simulink model "Proj4_sim"  (R2024b)
settings: Solver=VariableStepAuto  StartTime=0.0  StopTime=6000  RelTol=1e-3
values from neighbouring files (symbols this model uses):
  track_elevation_s = s_vals    [Proj4_track.m]
  track_elevation_z = elevation_profile    [Proj4_track.m]
undefined symbols (not defined in the file or in its folder): carData, datBat, datCar, datMotor, K_d, K_i, K_p
libraries: slpidlib x1, simulink x1
settings Model: NumberOfSteps=50  Creator=dxego  LastModifiedBy=jacobcody
settings RTWCC: GPUComputeCapability=3.5

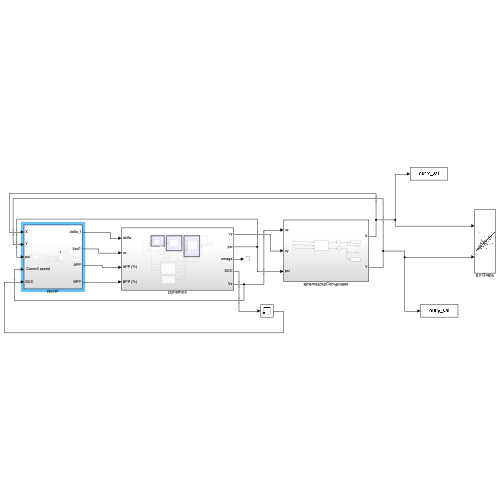
[thumbnail: Simulink's stored preview of the top-level diagram]
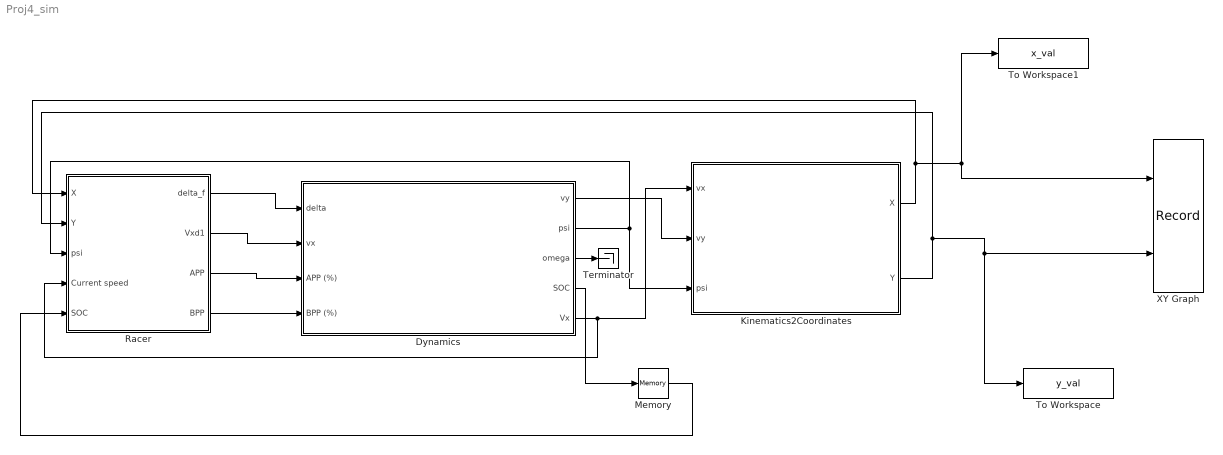
== system Proj4_sim ==
  Dynamics : Subsystem
  Kinematics2Coordinates : Subsystem
  Memory : Memory
  Racer : Subsystem
  Terminator : Terminator
  To Workspace : ToWorkspace  VariableName=y_val  SaveFormat=Timeseries  SampleTime=-1
  To Workspace1 : ToWorkspace  VariableName=x_val  SaveFormat=Timeseries  SampleTime=-1
  XY Graph : Record  FileSettingsInternal="{\"entries\":[{\"content\":{\"excelSettings\":{\"content\":{},\"type\":\"Streamout.ExcelSettings\"}},\"type\":\"Streamout.FileSettingStorage\",\"uuid\":\"\"}],\"packageUris\":[\"http:\\/\\/schema.mathworks.com\\/mf0\\/streamout_blocks\\/R2020a\"],\"version\":\"1.0\"}"  Layout=[1 1]  SignalsInternal="{\"entries\":[{\"content\":{\"signals\":[{\"content\":{\"blockPath\":[],\"dimensions\":[1],\"domain\":\"\",\"lineColor\":\"#ff13a6\",\"lineWidth\":2,\"port\":1,\"sid\":[\"\"],\"signalID\":1,\"signalName\":\"Kinematics2Coordinates:1\"},\"type\":\"RecordBlkView.Signal\",\"uuid\":\"\"},{\"content\":{\"blockPath\":[],\"dimensions\":[1],\"domain\":\"\",\"lineColor\":\"#139fff\",\"plots\":[ 1 ],\"port\":2,\"sid\":[\"\"],\"signalID\":2,\"signalName\":\"Kinematics2Coordinates:2\"},\"type\":\"RecordBlkView.Signal\",\"uuid\":\"\"}]},\"type\":\"RecordBlkView.InputSignals\",\"uuid\":\"\"}],\"packageUris\":[\"http:\\/\\/schema.mathworks.com\\/mf0\\/streamout_blocks\\/R2020a\"],\"version\":\"1.0\"}"  VisualizationBindings="{\"xyplotplugin\":{\"info\":[{\"series\":[{\"bindingParametersList\":[{\"parameter\":\"Y-Axis\",\"signalID\":2,\"signalName\":\"Kinematics2Coordinates:2\"}],\"seriesID\":0}],\"subplotID\":1}]}}"  CompatibilityTag=XY
  wires:
  Dynamics/1(vy) -> Kinematics2Coordinates/2(vy)
  Kinematics2Coordinates/1(X) -> Racer/1(X), To Workspace1/1, XY Graph/1
  Kinematics2Coordinates/2(Y) -> Racer/2(Y), To Workspace/1, XY Graph/2
  Racer/2(Vxd1) -> Dynamics/2(vx)
  Racer/1(delta_f) -> Dynamics/1(delta)
  Dynamics/2(psi) -> Kinematics2Coordinates/3(psi), Racer/3(psi)
  Dynamics/3(omega) -> Terminator/1
  Racer/3(APP) -> Dynamics/3(APP (%))
  Racer/4(BPP) -> Dynamics/4(BPP (%))
  Dynamics/5(Vx) -> Kinematics2Coordinates/1(vx), Racer/4(" Current speed")
  Memory/1 -> Racer/5("SOC ")
  Dynamics/4(SOC) -> Memory/1

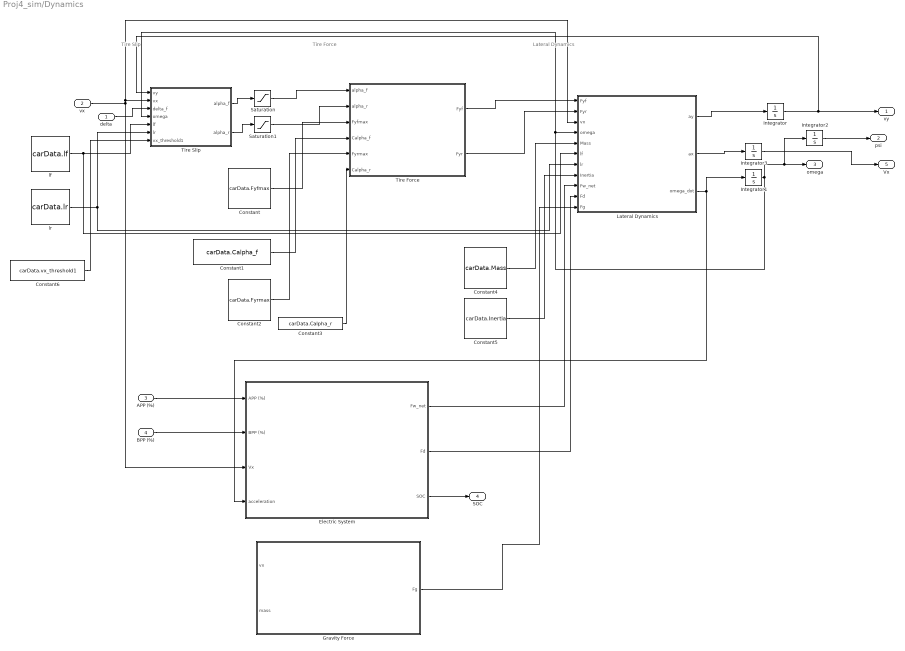
== system Proj4_sim/Dynamics ==
  note: Tire Slip
  note: Tire Force
  note: Lateral Dynamics
  delta : Inport
  vx : Inport  Port=2
  APP (%) : Inport  Port=3
  BPP (%) : Inport  Port=4
  Constant : Constant  Value=carData.Fyfmax
  Constant1 : Constant  Value=carData.Calpha_f
  Constant2 : Constant  Value=carData.Fyrmax
  Constant3 : Constant  Value=carData.Calpha_r
  Constant4 : Constant  Value=carData.Mass
  Constant5 : Constant  Value=carData.Inertia
  Constant6 : Constant  Value=carData.vx_threshold1
  Electric System : Subsystem
  Gravity Force : Subsystem
  Integrator : Integrator  InitialCondition=carData.init.vy0
  Integrator1 : Integrator  InitialCondition=carData.init.omega0
  Integrator2 : Integrator  InitialCondition=carData.init.psi0  WrappedStateUpperValue=2*pi  WrappedStateLowerValue=0
  Integrator3 : Integrator  InitialCondition=.01  IgnoreLimit=on
  Lateral Dynamics : MATLAB Function  TreatAsAtomicUnit=on
  Saturation : Saturate  UpperLimit=carData.maxAlpha  LowerLimit=-carData.maxAlpha
  Saturation1 : Saturate  UpperLimit=carData.maxAlpha  LowerLimit=-carData.maxAlpha
  Tire Force : MATLAB Function  TreatAsAtomicUnit=on
  "Tire Slip " : MATLAB Function  TreatAsAtomicUnit=on
  lf : Constant  Value=carData.lf
  lr : Constant  Value=carData.lr
  vy : Outport
  psi : Outport  Port=2
  omega : Outport  Port=3
  SOC : Outport  Port=4
  Vx : Outport  Port=5
  wires:
  Lateral Dynamics/1(ay) -> Integrator/1
  Integrator/1 -> "Tire Slip "/1(vy), vy/1
  Lateral Dynamics/3(omega_dot) -> Integrator1/1, Electric System/4(acceleration)
  Integrator1/1 -> Integrator2/1, omega/1, "Tire Slip "/4(omega), Lateral Dynamics/4(omega)
  "Tire Slip "/1(alpha_f) -> Saturation/1
  Saturation/1 -> Tire Force/1(alpha_f)
  Saturation1/1 -> Tire Force/2(alpha_r)
  vx/1 -> Lateral Dynamics/3(vx), "Tire Slip "/2(vx), Electric System/3(Vx)
  delta/1 -> "Tire Slip "/3(delta_f)
  Integrator2/1 -> psi/1
  "Tire Slip "/2(alpha_r) -> Saturation1/1
  Tire Force/1(Fyf) -> Lateral Dynamics/1(Fyf)
  Tire Force/2(Fyr) -> Lateral Dynamics/2(Fyr)
  lf/1 -> Lateral Dynamics/6(lf), "Tire Slip "/5(lf)
  lr/1 -> Lateral Dynamics/7(lr), "Tire Slip "/6(lr)
  Constant/1 -> Tire Force/3(Fyfmax)
  Constant1/1 -> Tire Force/4(Calpha_f)
  Constant2/1 -> Tire Force/5(Fyrmax)
  Constant3/1 -> Tire Force/6(Calpha_r)
  Constant4/1 -> Lateral Dynamics/5(Mass)
  Constant5/1 -> Lateral Dynamics/8(Inertia)
  Constant6/1 -> "Tire Slip "/7(vx_threshold1)
  APP (%)/1 -> Electric System/1(APP (%))
  BPP (%)/1 -> Electric System/2(BPP (%))
  Electric System/3(SOC) -> SOC/1
  Lateral Dynamics/2(ax) -> Integrator3/1
  Integrator3/1 -> Vx/1
  Electric System/2(Fd) -> Lateral Dynamics/10(Fd)
  Gravity Force/1(Fg) -> Lateral Dynamics/11(Fg)
  Electric System/1(Fw_net) -> Lateral Dynamics/9(Fw_net)

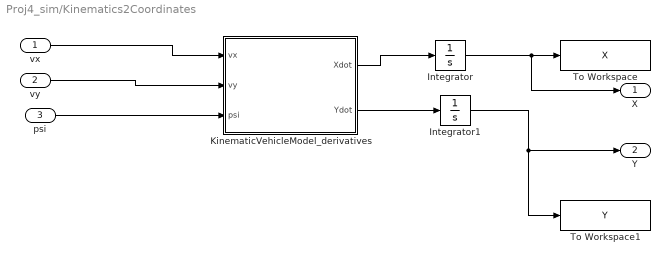
== system Proj4_sim/Kinematics2Coordinates ==
  vx : Inport
  vy : Inport  Port=2
  psi : Inport  Port=3
  Integrator : Integrator  InitialCondition=carData.init.X0
  Integrator1 : Integrator  InitialCondition=carData.init.Y0
  KinematicVehicleModel_derivatives : MATLAB Function  TreatAsAtomicUnit=on
  To Workspace : ToWorkspace  VariableName=X  SaveFormat=Timeseries  SampleTime=-1
  To Workspace1 : ToWorkspace  VariableName=Y  SaveFormat=Timeseries  SampleTime=-1
  X : Outport
  Y : Outport  Port=2
  wires:
  Integrator/1 -> X/1, To Workspace/1
  Integrator1/1 -> To Workspace1/1, Y/1
  vx/1 -> KinematicVehicleModel_derivatives/1(vx)
  vy/1 -> KinematicVehicleModel_derivatives/2(vy)
  psi/1 -> KinematicVehicleModel_derivatives/3(psi)
  KinematicVehicleModel_derivatives/1(Xdot) -> Integrator/1
  KinematicVehicleModel_derivatives/2(Ydot) -> Integrator1/1

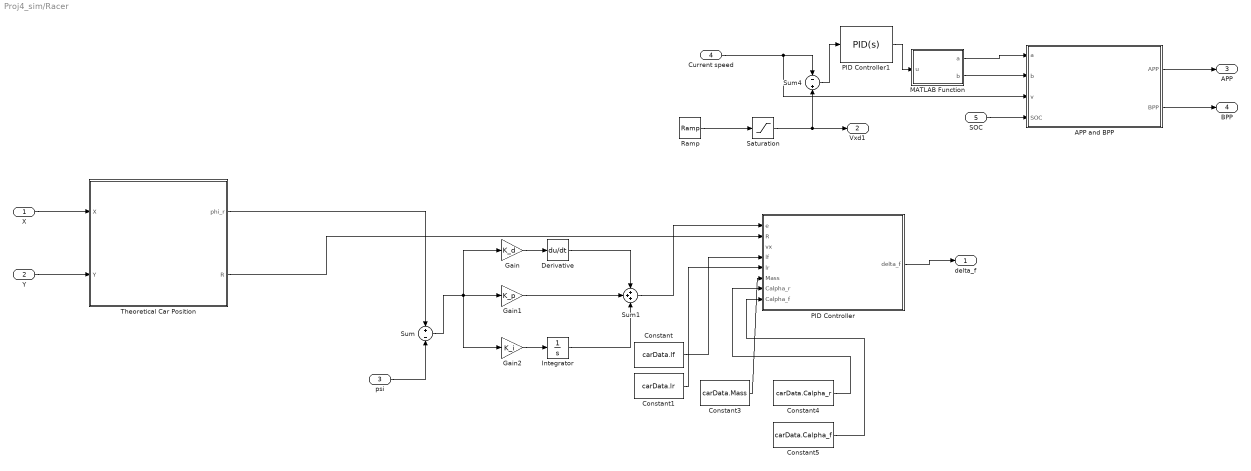
== system Proj4_sim/Racer ==
  X : Inport
  Y : Inport  Port=2
  psi : Inport  Port=3
  " Current speed" : Inport  Port=4
  "SOC " : Inport  Port=5
  "APP and BPP " : MATLAB Function  TreatAsAtomicUnit=on
  Constant : Constant  Value=carData.lf
  Constant1 : Constant  Value=carData.lr
  Constant3 : Constant  Value=carData.Mass
  Constant4 : Constant  Value=carData.Calpha_r
  Constant5 : Constant  Value=carData.Calpha_f
  Derivative : Derivative
  Gain : Gain  Gain=K_d
  Gain1 : Gain  Gain=K_p
  Gain2 : Gain  Gain=K_i
  Integrator : Integrator
  MATLAB Function : MATLAB Function  TreatAsAtomicUnit=on
  PID Controller : MATLAB Function  TreatAsAtomicUnit=on
  PID Controller1 : slpidlib/PID Controller  Controller=PID  Form=Parallel  TimeDomain=Continuous-time  UseExternalTs=off  SampleTime=-1  IntegratorMethod=Forward Euler  FilterMethod=Forward Euler  ControllerParametersSource=internal  P=2  I=0.8  UseKiTs=off  D=0  UseExternalDerivativeSource=off  N=100  UseFilter=on  TunerSelectOption=Transfer Function Based (PID Tuner App)  InitialConditionSource=internal  InitialConditionForIntegrator=0  InitialConditionForFilter=0  DifferentiatorICPrevScaledInput=0  ExternalReset=none  TrackingMode=off  Kt=1  LimitOutput=off  SatLimitsSource=internal  UpperSaturationLimit=inf  LowerSaturationLimit=-inf  LinearizeAsGain=on  AntiWindupMode=none  Kb=1  LimitIntegrator=off  UpperIntegratorSaturationLimit=inf  LowerIntegratorSaturationLimit=-inf  POutMin=[]  POutMax=[]  IOutMin=[]  IOutMax=[]  DOutMin=[]  DOutMax=[]  NOutMin=[]  NOutMax=[]  SumOutMin=[]  SumOutMax=[]  SaturationOutMin=[]  SaturationOutMax=[]  PParamMin=[]  PParamMax=[]  IParamMin=[]  IParamMax=[]  DParamMin=[]  DParamMax=[]  NParamMin=[]  NParamMax=[]  KbParamMin=[]  KbParamMax=[]  KtParamMin=[]  KtParamMax=[]  KbOutMin=[]  KbOutMax=[]  KtOutMin=[]  KtOutMax=[]  IntegratorOutMin=[]  IntegratorOutMax=[]  FilterOutMin=[]  FilterOutMax=[]  SumI1OutMin=[]  SumI1OutMax=[]  SumI2OutMin=[]  SumI2OutMax=[]  SumI3OutMin=[]  SumI3OutMax=[]  SumI4OutMin=[]  SumI4OutMax=[]  SumDOutMin=[]  SumDOutMax=[]  DifferentiatorOutMin=[]  DifferentiatorOutMax=[]  FilterDiffOutCoefMin=[]  FilterDiffOutCoefMax=[]  ReciprocalOutMin=[]  ReciprocalOutMax=[]  SumDenOutMin=[]  SumDenOutMax=[]  SumNumOutMin=[]  SumNumOutMax=[]  DivideOutMin=[]  DivideOutMax=[]  UdiffTsProdOutMin=[]  UdiffTsProdOutMax=[]  NTsProdOutMin=[]  NTsProdOutMax=[]  UintegralTsProdOutMin=[]  UintegralTsProdOutMax=[]  UngainTsProdOutMin=[]  UngainTsProdOutMax=[]  ClampingZeroOutDataTypeStr=Inherit: Inherit via back propagation  ClampingZeroOutMin=[]  ClampingZeroOutMax=[]  FilterDenConstantOutDataTypeStr=Inherit: Inherit via back propagation  FilterDenConstantOutMin=[]  FilterDenConstantOutMax=[]  PCopyOutDataTypeStr=Inherit: Inherit via back propagation  PCopyOutMin=[]  PCopyOutMax=[]  NCopyOutDataTypeStr=Inherit: Inherit via back propagation  NCopyOutMin=[]  NCopyOutMax=[]  IntegratorContinuousStateAttributes=''  IntegratorStateMustResolveToSignalObject=off  IntegratorRTWStateStorageClass=Auto  FilterContinuousStateAttributes=''  FilterStateMustResolveToSignalObject=off  FilterRTWStateStorageClass=Auto  ParallelPVariant=InternalParameters  IdealPVariant=Disabled  IVariant=InternalParameters  DVariant=InternalParameters  IntegratorVariant=Continuous  SatVariant=Disabled  AWVariant=Passthrough  PCopyVariant=Disabled  TRVariant=Disabled  FdbkBlocksVariant=Forward  IdealPFdbkVariant=Disabled  SatFdbkVariant=Disabled  DerivativeFilterVariant=ContFilter  NVariant=InternalParameters  NCopyVariant=Disabled  FilterICVariant=InternalICsFilter  IntegratorICVariant=InternalICs  ExternalResetVariant=Disabled  TRSumVariant=Passthrough  SumFdbkVariant=Disabled  SumVariant=Sum_PID  TsampFilterVariant=InternalTs  TsampNgainVariant=Passthrough  TsampIntegralVariant=Disabled_SignalSpec  ExternalSaturationOutDataTypeStr=Inherit: Same as second input  DerivativeSourceVariant=ErrorSignal  PreIntVariant=InternalPreInt
  Ramp : simulink/Sources/Ramp  slope=2.5  start=0  InitialOutput=0
  Saturation : Saturate  UpperLimit=10  LowerLimit=0
  Sum : Sum  Inputs=+-
  Sum1 : Sum  Inputs=+++
  Sum4 : Sum  Inputs=-+
  Theoretical Car Position : MATLAB Function  TreatAsAtomicUnit=on
  delta_f : Outport
  Vxd1 : Outport  Port=2
  APP : Outport  Port=3
  BPP : Outport  Port=4
  wires:
  Y/1 -> Theoretical Car Position/2(Y)
  psi/1 -> Sum/2
  Gain/1 -> Derivative/1
  Gain2/1 -> Integrator/1
  Sum/1 -> Gain2/1, Gain/1, Gain1/1
  Derivative/1 -> Sum1/1
  Gain1/1 -> Sum1/2
  Integrator/1 -> Sum1/3
  Sum1/1 -> PID Controller/1(e)
  X/1 -> Theoretical Car Position/1(X)
  Constant/1 -> PID Controller/4(lf)
  Constant1/1 -> PID Controller/5(lr)
  Constant3/1 -> PID Controller/6(Mass)
  Constant4/1 -> PID Controller/7(Calpha_r)
  Constant5/1 -> PID Controller/8(Calpha_f)
  Theoretical Car Position/1(phi_r) -> Sum/1
  Theoretical Car Position/2(R) -> PID Controller/2(R)
  PID Controller/1(delta_f) -> delta_f/1
  Ramp/1 -> Saturation/1
  "APP and BPP "/1(APP) -> APP/1
  "APP and BPP "/2(BPP) -> BPP/1
  "SOC "/1 -> "APP and BPP "/4(SOC)
  " Current speed"/1 -> "APP and BPP "/3(v), Sum4/1
  Saturation/1 -> Vxd1/1, Sum4/2
  Sum4/1 -> PID Controller1/1
  PID Controller1/1 -> MATLAB Function/1(u)
  MATLAB Function/1(a) -> "APP and BPP "/1(a)
  MATLAB Function/2(b) -> "APP and BPP "/2(b)

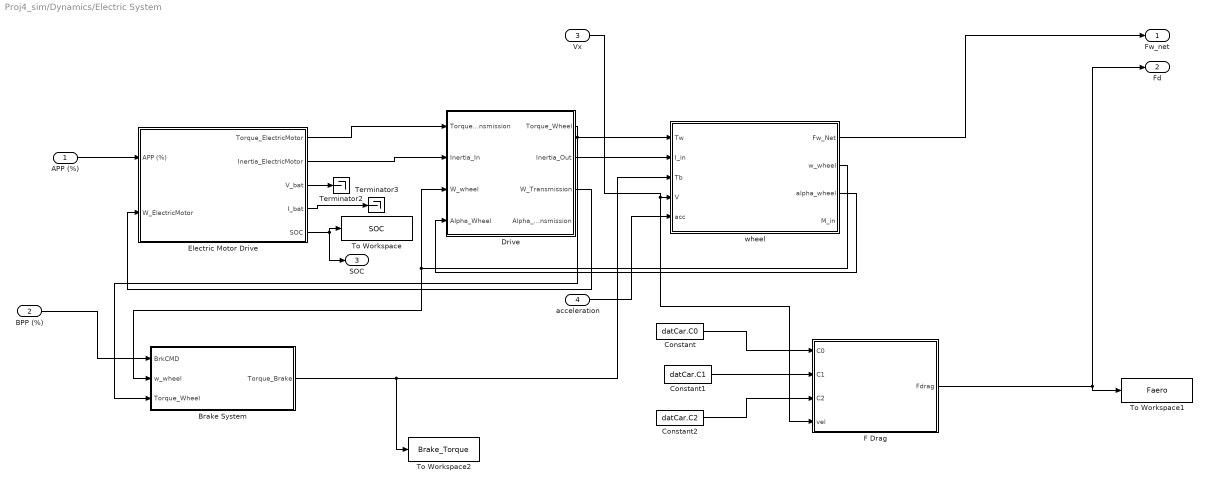
== system Proj4_sim/Dynamics/Electric System ==
  APP (%) : Inport
  BPP (%) : Inport  Port=2
  Vx : Inport  Port=3
  acceleration : Inport  Port=4
  "Brake System " : Subsystem
  Constant : Constant  Value=datCar.C0
  Constant1 : Constant  Value=datCar.C1
  Constant2 : Constant  Value=datCar.C2
  Drive : Subsystem
  Electric Motor Drive : Subsystem
  F Drag : MATLAB Function  TreatAsAtomicUnit=on
  Terminator2 : Terminator
  Terminator3 : Terminator
  To Workspace : ToWorkspace  VariableName=SOC  SaveFormat=Timeseries  SampleTime=-1
  To Workspace1 : ToWorkspace  VariableName=Faero  SaveFormat=Timeseries  SampleTime=-1
  To Workspace2 : ToWorkspace  VariableName=Brake_Torque  SaveFormat=Timeseries  SampleTime=-1
  "wheel " : Subsystem
  Fw_net : Outport
  Fd : Outport  Port=2
  SOC : Outport  Port=3
  wires:
  Drive/2(Inertia_Out) -> "wheel "/2(I_in)
  Vx/1 -> F Drag/4(vel), "wheel "/4(V)
  Drive/1(Torque_Wheel) -> "Brake System "/3(Torque_Wheel), "wheel "/1(Tw)
  APP (%)/1 -> Electric Motor Drive/1(APP (%))
  Electric Motor Drive/1(Torque_ElectricMotor) -> Drive/1(Torque_Transmission)
  Electric Motor Drive/2(Inertia_ElectricMotor) -> Drive/2(Inertia_In)
  Electric Motor Drive/3(V_bat) -> Terminator2/1
  Electric Motor Drive/4(I_bat) -> Terminator3/1
  Electric Motor Drive/5(SOC) -> To Workspace/1, SOC/1
  acceleration/1 -> "wheel "/5(acc)
  "wheel "/1(Fw_Net) -> Fw_net/1
  F Drag/1(Fdrag) -> To Workspace1/1, Fd/1
  BPP (%)/1 -> "Brake System "/1("BrkCMD ")
  "wheel "/3(alpha_wheel) -> Drive/4(Alpha_Wheel)
  "wheel "/2(w_wheel) -> Drive/3(W_wheel), "Brake System "/2("w_wheel ")
  Constant/1 -> F Drag/1(C0)
  Constant1/1 -> F Drag/2(C1)
  Constant2/1 -> F Drag/3(C2)
  "Brake System "/1("Torque_Brake ") -> To Workspace2/1, "wheel "/3(Tb)
  Drive/3(W_Transmission) -> Electric Motor Drive/2(W_ElectricMotor)

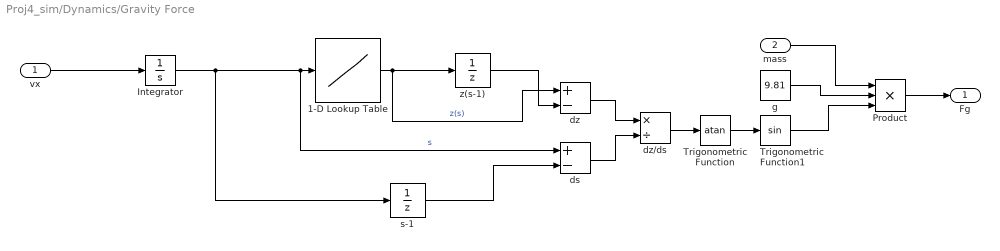
== system Proj4_sim/Dynamics/Gravity Force ==
  vx : Inport
  mass : Inport  Port=2
  1-D Lookup Table : Lookup_n-D  NumberOfTableDimensions=1  BreakpointsForDimension1=track_elevation_s  Table=track_elevation_z  InternalRulePriority=Speed  RndMeth=Simplest
  Integrator : Integrator
  Product : Product  Inputs=3
  Trigonometric Function : Trigonometry  Operator=atan
  Trigonometric Function1 : Trigonometry
  ds : Sum  Inputs=+-
  dz : Sum  Inputs=+-
  dz/ds : Product  Inputs=*/
  g : Constant  Value=9.81
  s-1 : UnitDelay  SampleTime=-1  HasFrameUpgradeWarning=on
  z(s-1) : UnitDelay  SampleTime=-1  HasFrameUpgradeWarning=on
  Fg : Outport
  wires:
  vx/1 -> Integrator/1
  Integrator/1 -> s-1/1, ds/1, 1-D Lookup Table/1  "s"
  1-D Lookup Table/1 -> z(s-1)/1, dz/1  "z(s)"
  z(s-1)/1 -> dz/2
  dz/1 -> dz/ds/1
  ds/1 -> dz/ds/2
  dz/ds/1 -> Trigonometric Function/1
  Trigonometric Function/1 -> Trigonometric Function1/1
  mass/1 -> Product/1
  g/1 -> Product/2
  Trigonometric Function1/1 -> Product/3
  Product/1 -> Fg/1
  s-1/1 -> ds/2

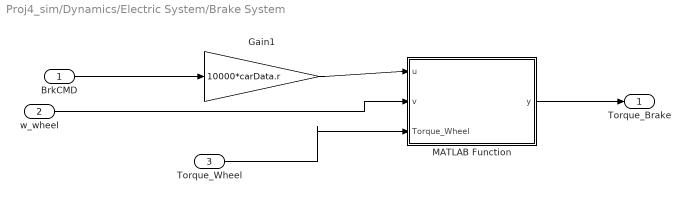
== system Proj4_sim/Dynamics/Electric System/Brake System  ==
  "BrkCMD " : Inport
  "w_wheel " : Inport  Port=2
  Torque_Wheel : Inport  Port=3
  Gain1 : Gain  Gain=10000*carData.r
  MATLAB Function : MATLAB Function  TreatAsAtomicUnit=on
  "Torque_Brake " : Outport  VectorParamsAs1DForOutWhenUnconnected=off
  wires:
  "BrkCMD "/1 -> Gain1/1
  Gain1/1 -> MATLAB Function/1(u)
  "w_wheel "/1 -> MATLAB Function/2(v)
  MATLAB Function/1(y) -> "Torque_Brake "/1
  Torque_Wheel/1 -> MATLAB Function/3(Torque_Wheel)

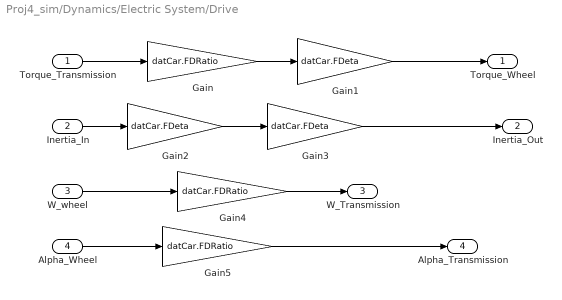
== system Proj4_sim/Dynamics/Electric System/Drive ==
  Torque_Transmission : Inport
  Inertia_In : Inport  Port=2
  W_wheel : Inport  Port=3
  Alpha_Wheel : Inport  Port=4
  Gain : Gain  Gain=datCar.FDRatio
  Gain1 : Gain  Gain=datCar.FDeta
  Gain2 : Gain  Gain=datCar.FDeta
  Gain3 : Gain  Gain=datCar.FDeta
  Gain4 : Gain  Gain=datCar.FDRatio
  Gain5 : Gain  Gain=datCar.FDRatio
  Torque_Wheel : Outport
  Inertia_Out : Outport  Port=2
  W_Transmission : Outport  Port=3
  Alpha_Transmission : Outport  Port=4
  wires:
  Torque_Transmission/1 -> Gain/1
  Gain/1 -> Gain1/1
  Gain1/1 -> Torque_Wheel/1
  Inertia_In/1 -> Gain2/1
  Gain2/1 -> Gain3/1
  Gain3/1 -> Inertia_Out/1
  W_wheel/1 -> Gain4/1
  Gain4/1 -> W_Transmission/1
  Alpha_Wheel/1 -> Gain5/1
  Gain5/1 -> Alpha_Transmission/1

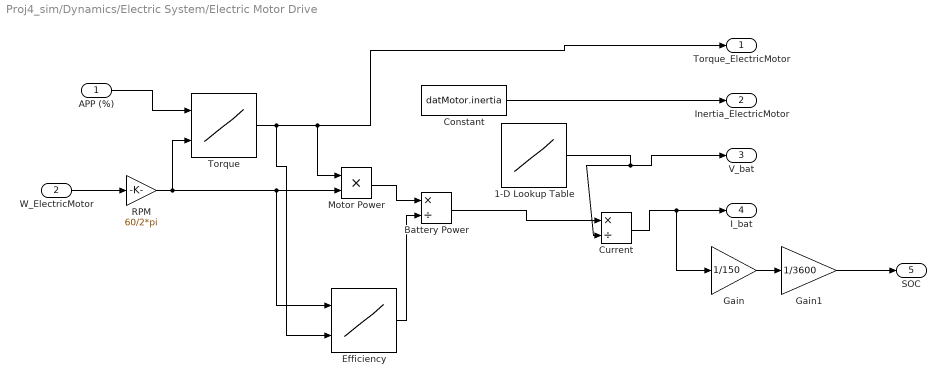
== system Proj4_sim/Dynamics/Electric System/Electric Motor Drive ==
  APP (%) : Inport
  W_ElectricMotor : Inport  Port=2
  1-D Lookup Table : Lookup_n-D  NumberOfTableDimensions=1  BreakpointsForDimension1=datBat.SOC  Table=datBat.OCV * datBat.numSeries  InternalRulePriority=Speed  RndMeth=Simplest
  Battery Power : Product  Inputs=*/
  Constant : Constant  Value=datMotor.inertia
  Current : Product  Inputs=*/
  Efficiency : Lookup_n-D  BreakpointsForDimension1=datMotor.eta_torque  BreakpointsForDimension2=datMotor.eta_speed  Table=datMotor.eta_val  InternalRulePriority=Speed  RndMeth=Simplest
      settings: InputPortMap=u0,u1
  Gain : Gain  Gain=1/150
  Gain1 : Gain  Gain=1/3600
  Motor Power : Product
  RPM : Gain  Gain=60/2*pi
  Torque : Lookup_n-D  BreakpointsForDimension1=[0,25,50,75,100]  BreakpointsForDimension2=datMotor.rpm  Table=datMotor.maxtorque  InternalRulePriority=Speed  RndMeth=Simplest
      settings: InputPortMap=u0,u1
  Torque_ElectricMotor : Outport
  Inertia_ElectricMotor : Outport  Port=2
  V_bat : Outport  Port=3
  I_bat : Outport  Port=4
  SOC : Outport  Port=5
  wires:
  Battery Power/1 -> Current/1
  1-D Lookup Table/1 -> Current/2, V_bat/1
  W_ElectricMotor/1 -> RPM/1
  APP (%)/1 -> Torque/1
  Constant/1 -> Inertia_ElectricMotor/1
  Torque/1 -> Efficiency/2, Torque_ElectricMotor/1, Motor Power/1
  Motor Power/1 -> Battery Power/1
  Efficiency/1 -> Battery Power/2
  RPM/1 -> Efficiency/1, Motor Power/2, Torque/2
  Current/1 -> Gain/1, I_bat/1
  Gain/1 -> Gain1/1
  Gain1/1 -> SOC/1

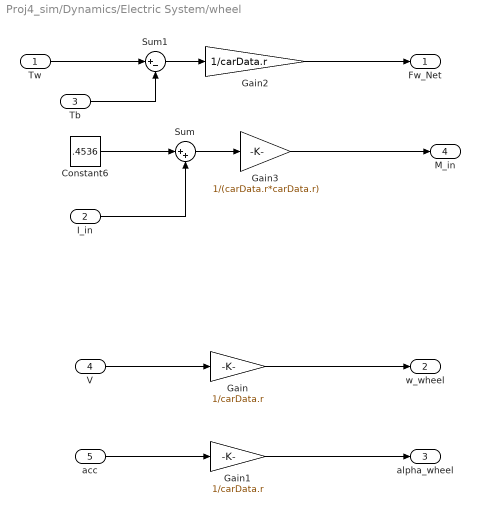
== system Proj4_sim/Dynamics/Electric System/wheel  ==
  Tw : Inport
  I_in : Inport  Port=2
  Tb : Inport  Port=3
  V : Inport  Port=4
  acc : Inport  Port=5
  Constant6 : Constant  Value=.4536
  Gain : Gain  Gain=1/carData.r
  Gain1 : Gain  Gain=1/carData.r
  Gain2 : Gain  Gain=1/carData.r
  Gain3 : Gain  Gain=1/(carData.r*carData.r)
  Sum : Sum  Inputs=|++
  Sum1 : Sum  Inputs=|+-
  Fw_Net : Outport
  w_wheel : Outport  Port=2
  alpha_wheel : Outport  Port=3
  M_in : Outport  Port=4
  wires:
  Gain/1 -> w_wheel/1
  V/1 -> Gain/1
  acc/1 -> Gain1/1
  Gain1/1 -> alpha_wheel/1
  Gain2/1 -> Fw_Net/1
  Constant6/1 -> Sum/1
  I_in/1 -> Sum/2
  Sum/1 -> Gain3/1
  Gain3/1 -> M_in/1
  Tw/1 -> Sum1/1
  Tb/1 -> Sum1/2
  Sum1/1 -> Gain2/1

== matlab function Proj4_sim/Racer/PID Controller ==
  data: e input; delta_f output; R input; vx input; lf input; lr input; Mass input; Calpha_r input; Calpha_f input
function delta_f = fcn(e, R, vx, lf, lr, Mass, Calpha_r, Calpha_f)
L = lr + lf;
if R ~= 0
    delta_f = e + (L/R)+((Mass/(L*R))*((lr/Calpha_r)-(lf/Calpha_f))*(vx^2));
else
    delta_f = e;

end

== matlab function Proj4_sim/Racer/APP and BPP  ==
  data: a input; b input; APP output; BPP output; v input; SOC input
function [APP, BPP] = fcn(a, b, v, SOC)

mph2mps = 1600/3600; % mph to m/s conversion
V_low = 5 * mph2mps;   
V_high = 25 * mph2mps; 

%Initialize
APP = 0;
BPP = 0;

if b > 0 %If braking is requested
    if v <= V_low
        FrictionPercent = 1; %100% friction
    elseif v < V_high
        FrictionPercent = 1 - 0.95 * (v - V_low) / (V_high - V_low);
    else
        FrictionPercent = 0.05; %5% friction
    end

    RegenPercent = 1 - FrictionPercent;

    if SOC <= 0.1
        RegenPercent = 0;
        FrictionPercent = 1;
    end
    APP = a + b * RegenPercent; %Add regen to throttle
    BPP = b * FrictionPercent;  %Only friction goes to brake pedal

else
    %No braking, normal acceleration
    APP = a;
    BPP = 0;
end

end

== matlab function Proj4_sim/Racer/MATLAB Function ==
  data: u input; a output; b output
function [a, b] = fcn(u)

if u >= 0
    a = min(u, 100); 
    b = 0;           
else
    a = 0;           
    b = min(-u, 100);
end

end

== matlab function Proj4_sim/Dynamics/Electric System/F Drag ==
  data: C0 input; Fdrag output; C1 input; C2 input; vel input
function Fdrag = fcn(C0,C1,C2,vel)

Fdrag = C0 + C1*vel + C2*vel^2;

== matlab function Proj4_sim/Dynamics/Tire Slip  ==
  data: vy input; alpha_f output; vx input; delta_f input; omega input; lf input; alpha_r output; lr input; vx_threshold1 input
function [alpha_f, alpha_r] = fcn(vy,  vx, delta_f, omega, lf, lr, vx_threshold1)


if abs(vx)> vx_threshold1
      alpha_f = delta_f - (vy + omega * lf) / vx;
      alpha_r = - (vy - omega * lr) / vx;
else
      alpha_f = 0;
      alpha_r = 0;
end



end

== matlab function Proj4_sim/Racer/Theoretical Car Position ==
  data: X input; phi_r output; Y input; R output
function [phi_r, R] = car_position(X, Y)

    phi_r = 0;
    R = 0;

    if Y < 200
        if X >= 0 && X <= 900
            phi_r = 0; % first straight path from origin
            R = 0;
        elseif X > 900
            val = (X - 900) / 200;
            val = min(max(val, -1), 1); 
            phi_r = 2*pi - acos(val) - deg2rad(270); % first turn
            R = 200;
        elseif X < 0
            val = (-X) / 200;
            val = min(max(val, -1), 1); 
            phi_r = acos(val) + deg2rad(270); % turn 4
            R = 200;
        end
    else
        if X >= 0 && X <= 900
            phi_r = pi; % second straight path
            R = 0;
        elseif X > 900
            val = (X - 900) / 200;
            val = min(max(val, -1), 1); 
            phi_r = acos(val) + deg2rad(90); % turn 2
            R = 200;
        elseif X < 0
            val = (-X) / 200;
            val = min(max(val, -1), 1); 
            phi_r = 2*pi - acos(val) - deg2rad(90); % turn 3
            R = 200;
        end
    end

end

== matlab function Proj4_sim/Dynamics/Electric System/Brake System /MATLAB Function ==
  data: u input; y output; v input; Torque_Wheel input
function y = fcn(u,v,Torque_Wheel)
    y_brake = u * v / (abs(v) + 0.001);  
    y = y_brake - Torque_Wheel;
    
    if y < 0
        y = 0;
    end
end

== matlab function Proj4_sim/Kinematics2Coordinates/KinematicVehicleModel_derivatives ==
  data: vx input; Xdot output; vy input; psi input; Ydot output
function [Xdot, Ydot] = fcn(vx, vy, psi)
    temp = TF(psi) * [vx;vy]; 
    Xdot = temp(1);
    Ydot = temp(2);
  
end

function y = TF(psi)
    y = [cos(psi), -sin(psi); sin(psi), cos(psi)];
end

== matlab function Proj4_sim/Dynamics/Tire Force ==
  data: alpha_f input; Fyf output; alpha_r input; Fyfmax input; Fyr output; Calpha_f input; Fyrmax input; Calpha_r input
function [Fyf, Fyr] = fcn(alpha_f, alpha_r, Fyfmax, Calpha_f, Fyrmax, Calpha_r)

Fyf = min(Fyfmax,Calpha_f * alpha_f);
Fyr = min(Fyrmax, Calpha_r * alpha_r);

end

== matlab function Proj4_sim/Dynamics/Lateral Dynamics ==
  data: Fyf input; ay output; ax output; Fyr input; vx input; omega input; Mass input; omega_dot output; lf input; lr input; Inertia input; Fw_net input; Fd input; Fg input
function [ay, ax, omega_dot] = fcn(Fyf, Fyr, vx, omega, Mass, lf, lr, Inertia, Fw_net, Fd,Fg)
Fy = Fyf + Fyr;
ay = Fy / Mass - omega * vx;
        
M  = Fyf * lf - Fyr *lr;        
omega_dot = M / Inertia;

Fx = Fw_net - Fd%-Fg;

ax= Fx/Mass;
end
